simulink model "distance"  (R2018b)
settings: Solver=FixedStepAuto  StartTime=0.0  StopTime=10  FixedStep=continuous_h  RelTol=1e-3
StopFcn:
  | plot3_state
undefined symbols (not defined in the file or in its folder): continuous_h, distc_params, traj
libraries: simulink x3, cf_lib x1, vel_controller_lib x1
settings Model: Creator=Pontus  LastModifiedBy=Pontus
settings OptimizationCC: DefaultParameterBehavior=Inlined  UseFloatMulNetSlope=on  InlineInvariantSignals=on  PassReuseOutputArgsAs=Individual arguments  ZeroExternalMemoryAtStartup=off  ZeroInternalMemoryAtStartup=off  NoFixptDivByZeroProtection=on  EfficientFloat2IntCast=on  LifeSpan=1  OptimizeBlockOrder=speed  DifferentSizesBufferReuse=on
settings DebuggingCC: ParameterTunabilityLossMsg=error
settings HardwareCC: ProdLongLongMode=on
settings SFSimCC: MATLABDynamicMemAlloc=off
settings RTWCC: SystemTargetFile=ert.tlc  TemplateMakefile=ert_default_tmf  GenerateReport=on  IncludeHyperlinkInReport=on  LaunchReport=on  GenerateTraceInfo=on  GenerateTraceReport=on  GenerateTraceReportSl=on  GenerateTraceReportSf=on  GenerateTraceReportEml=on  GenerateCodeMetricsReport=on
settings CodeAppCC: ForceParamTrailComments=on  IgnoreCustomStorageClasses=off  OperatorAnnotations=on  SimulinkDataObjDesc=on  SFDataObjDesc=on  InsertBlockDesc=on
settings ERTTargetCC: TargetLangStandard=C99 (ISO)  GenerateSampleERTMain=on  IncludeMdlTerminateFcn=off  CombineSignalStateStructs=on  SupportComplex=off  SupportNonInlinedSFcns=on  InlinedParameterPlacement=NonHierarchical  ERTCustomFileTemplate=example_file_process.tlc  ERTFilePackagingFormat=CompactWithDataFile

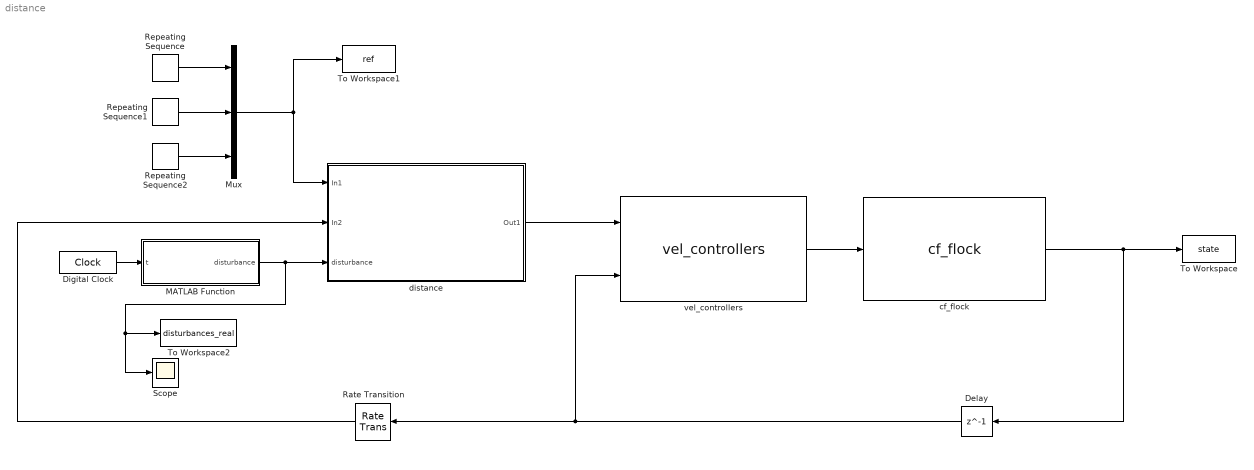
== system distance ==
  Delay : Delay  DelayLength=1
  Digital Clock : DigitalClock  SampleTime=continuous_h
  MATLAB Function : MATLAB Function  TreatAsAtomicUnit=on
  Mux : Mux  Inputs=3
  Rate Transition : RateTransition  OutPortSampleTime=0.05
  Repeating Sequence : simulink/Sources/Repeating Sequence  rep_seq_t=traj.seq_t  rep_seq_y=traj.seq(1,:)
  Repeating Sequence1 : simulink/Sources/Repeating Sequence  rep_seq_t=traj.seq_t  rep_seq_y=traj.seq(2,:)
  Repeating Sequence2 : simulink/Sources/Repeating Sequence  rep_seq_t=traj.seq_t  rep_seq_y=traj.seq(3,:)
  Scope : Scope
  To Workspace : ToWorkspace  VariableName=state  SaveFormat=Timeseries  SampleTime=-1
  To Workspace1 : ToWorkspace  VariableName=ref  SaveFormat=Timeseries  SampleTime=continuous_h
  To Workspace2 : ToWorkspace  VariableName=disturbances_real  SaveFormat=Timeseries  SampleTime=-1
  cf_flock : cf_lib/cf_flock  SystemSampleTime=-1
  distance : Subsystem
  vel_controllers : vel_controller_lib/vel_controllers  SystemSampleTime=-1
      link override vel_controller/Transport Delay: DelayTime=0.005
  wires:
  Delay/1 -> Rate Transition/1, vel_controllers/2
  Mux/1 -> distance/1(In1), To Workspace1/1
  cf_flock/1 -> To Workspace/1, Delay/1
  Repeating Sequence/1 -> Mux/1
  Repeating Sequence1/1 -> Mux/2
  Repeating Sequence2/1 -> Mux/3
  vel_controllers/1 -> cf_flock/1
  distance/1(Out1) -> vel_controllers/1
  MATLAB Function/1(disturbance) -> To Workspace2/1, Scope/1, distance/3(disturbance)
  Digital Clock/1 -> MATLAB Function/1(t)
  Rate Transition/1 -> distance/2(In2)

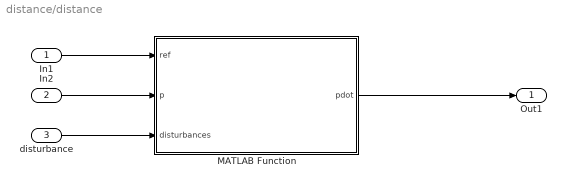
== system distance/distance ==
  In1 : Inport
  In2 : Inport  Port=2
  disturbance : Inport  Port=3
  MATLAB Function : MATLAB Function  TreatAsAtomicUnit=on  SystemSampleTime=distc_params.h
  Out1 : Outport
  wires:
  In2/1 -> MATLAB Function/2(p)
  In1/1 -> MATLAB Function/1(ref)
  MATLAB Function/1(pdot) -> Out1/1
  disturbance/1 -> MATLAB Function/3(disturbances)

== matlab function distance/MATLAB Function ==
  data: t input; disturbances parameter; disturbance output
function disturbance = dynamic_disturbance(t, disturbances)
disturbance = disturbances;
disturbance(3,1) = disturbances(3,1) - 49.6 + 30*t - 9.82*t^2/2;
disturbance(1,1) = disturbances(1,1) - 3 + 1*t;

== matlab function distance/MATLAB Function ==
  data: ref input; p input; pdot output; distc_params parameter; disturbances input
function pdot = distance_controller(ref,p,distc_params,disturbances)
% Calculate velocity vector pdot, from equation 4.4 in Zhiyong's
% thesis. Includes formation control as well as trajectory control
persistent integ prev_e_swarm;

if isempty(integ)
    integ = [0;0;0];
end
if isempty(prev_e_swarm)
    prev_e_swarm = [0;0;0];
end

p = p(1:3,:);
[~,c] = size(p);
pdot=zeros(size(p));
p_swarm = zeros(3,1);
[~,n_d] = size(disturbances);

for i=1:c
    p_swarm = p_swarm + p(1:3,i)/c; %Center position of swarm
end

%Calculate swarm ref error and corresponding integral/derivative parts 
e_swarm = ref - p_swarm;
integ = integ + distc_params.ki*distc_params.h*e_swarm;
deriv = (e_swarm - prev_e_swarm)*distc_params.kd/distc_params.h;

%Calculate desired velocity due to distance between drones
for i=1:c
    for j=1:c
        p_norm = max(norm(p(:,i)-p(:,j)),0.05); %Init with 5 cm
        p_norm2 = (p_norm-distc_params.d(i,j))/p_norm;
                
        pdot(:,i) = pdot(:,i) - (p(:,i)-p(:,j))*p_norm2;        
    end
    
    %Disturbance contribution
    for k=1:n_d    
        disturb_dist = [p(:,i) - disturbances(1:3,k); disturbances(4,k)];
        
        % Option 4 for distance controller
        [dir,magn] = calculate_disturbance(disturb_dist,4);
        
        pdot(:,i) = pdot(:,i) + magn*distc_params.kdisturb*dir;
    
    end
    
    %Add control signal from trajectory reference
    pdot(:,i) = pdot(:,i) + distc_params.kp*e_swarm + integ + deriv;
end

%Save error for next sample
prev_e_swarm = e_swarm;

end
